simulink model "SVPWM_simscape"  (R2026a)
settings: Solver=ode23t  StartTime=1  StopTime=2  FixedStep=1e-7  RelTol=1e-5  AbsTol=1e-10
undefined symbols (not defined in the file): Down, PermanentMagnetSynchrono_class, Up
libraries: fl_lib x24, nesl_utility x20, ee_lib x8, eeTransforms x4, eePwmGenerator x3, simulink x3, elec_conv_HighZElecRef x2
(part 1 of 2)
settings Model: SimulationMode=accelerator  Creator=刘炳宏  LastModifiedBy=mushen
settings DebuggingCC: SaveWithParameterizedLinksMsg=none
settings SimscapeCC: SimscapeLogType=none  SimscapeLogDataHistory=5000.0

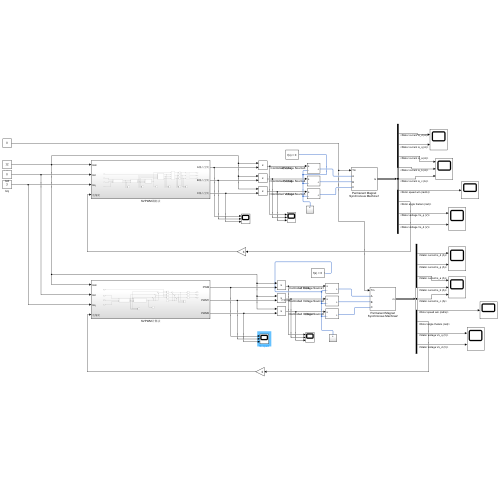
[thumbnail: Simulink's stored preview of the top-level diagram]
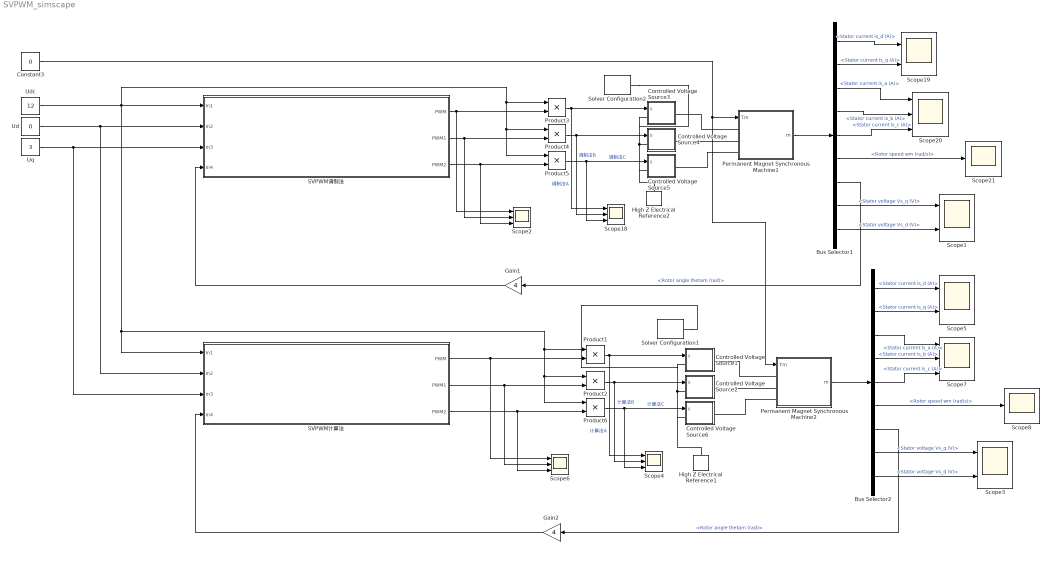
== system SVPWM_simscape ==
  Bus Selector1 : BusSelector  OutputSignals=Stator current is_d (A),Stator current is_q (A),Stator current is_a (A),Stator current is_b (A),Stator current is_c (A),Rotor speed wm (rad/s),Rotor angle thetam (rad),Stator voltage Vs_q (V),Stator voltage Vs_d (V)
  Bus Selector2 : BusSelector  OutputSignals=Stator current is_d (A),Stator current is_q (A),Stator current is_a (A),Stator current is_b (A),Stator current is_c (A),Rotor speed wm (rad/s),Rotor angle thetam (rad),Stator voltage Vs_q (V),Stator voltage Vs_d (V)
  Constant3 : Constant  Value=0
  Controlled Voltage Source1 : Subsystem
      settings: OpenFcn=elec.conv.unmask(gcb);
  Controlled Voltage Source2 : Subsystem
      settings: OpenFcn=elec.conv.unmask(gcb);
  Controlled Voltage Source3 : Subsystem
      settings: OpenFcn=elec.conv.unmask(gcb);
  Controlled Voltage Source4 : Subsystem
      settings: OpenFcn=elec.conv.unmask(gcb);
  Controlled Voltage Source5 : Subsystem
      settings: OpenFcn=elec.conv.unmask(gcb);
  Controlled Voltage Source6 : Subsystem
      settings: OpenFcn=elec.conv.unmask(gcb);
  Gain1 : Gain  Gain=4
  Gain2 : Gain  Gain=4
  High Z Electrical Reference1 : elec_conv_HighZElecRef/High Z Electrical Reference  SystemSampleTime=-1  VariantActivationTime=update diagram  EmptyChoice=off  PassThrough=off  PassThroughVariantControl=(default)  EmptyChoiceVariantControl=(default)  AllowFlexibleInterface=on  Latency=0  AutoFrameSizeCalculation=off
  High Z Electrical Reference2 : elec_conv_HighZElecRef/High Z Electrical Reference  SystemSampleTime=-1  VariantActivationTime=update diagram  EmptyChoice=off  PassThrough=off  PassThroughVariantControl=(default)  EmptyChoiceVariantControl=(default)  AllowFlexibleInterface=on  Latency=0  AutoFrameSizeCalculation=off
  Permanent Magnet Synchronous Machine1 : Subsystem
      settings: OpenFcn=elec.conv.unmask(gcb);
  Permanent Magnet Synchronous Machine2 : Subsystem
      settings: OpenFcn=elec.conv.unmask(gcb);
  Product{1..6} (6 alike) : Product
  SVPWM计算法 : Subsystem
  SVPWM调制法 : Subsystem
  Scope{1,3,5,19} (4 alike) : Scope  NumInputPorts=2
      Scope1 settings: ActiveDisplayYMinimum=-0.375  ActiveDisplayYMaximum=3.375
      Scope19 settings: ActiveDisplayYMinimum=-2.03311  ActiveDisplayYMaximum=2.45595  DataLoggingVariableName=ScopeData9
      Scope3 settings: ActiveDisplayYMinimum=-0.375  ActiveDisplayYMaximum=3.375  DataLoggingVariableName=ScopeData5
      Scope5 settings: ActiveDisplayYMinimum=-1.22545  ActiveDisplayYMaximum=3.73742  DataLoggingVariableName=ScopeData7
  Scope{2,4,6..7,18,20} (6 alike) : Scope  NumInputPorts=3
      Scope18 settings: ActiveDisplayYMinimum=2.7524  ActiveDisplayYMaximum=9.2476  DataLoggingVariableName=ScopeData8
      Scope2 settings: ActiveDisplayYMinimum=0.22937  ActiveDisplayYMaximum=0.77063
      Scope20 settings: ActiveDisplayYMinimum=-2.08518  ActiveDisplayYMaximum=2.2657  DataLoggingVariableName=ScopeData10
      Scope4 settings: ActiveDisplayYMinimum=-1.5  ActiveDisplayYMaximum=13.5  DataLoggingVariableName=ScopeData6
      Scope6 settings: ActiveDisplayYMinimum=0.22936706131906309  ActiveDisplayYMaximum=0.770632938680937  DataLoggingVariableName=ScopeData8
      Scope7 settings: ActiveDisplayYMinimum=-10.80387  ActiveDisplayYMaximum=10.80369  DataLoggingVariableName=ScopeData9
  Scope21 : Scope
      settings: ActiveDisplayYMinimum=-17.67923  ActiveDisplayYMaximum=27.92177  DataLoggingVariableName=ScopeData11
  Scope8 : Scope
      settings: ActiveDisplayYMinimum=-2.22769  ActiveDisplayYMaximum=20.0492  DataLoggingVariableName=ScopeData10
  Solver Configuration1 : nesl_utility/Solver Configuration  PhysicalDomain=network_engine_domain  SubClassName=solver  LeftPortType=input  RightPortType=generic  Tones=[]  Harmonics=[]  SimulateNoise=off  Profile=off  UseLocalSampling=off  EnableSwitchedLinearOptims=on  FrequencyDomain=off  UseCCode=off  RelTol=0.001  AbsTol=0.001  MinStep=1e-09  ToWorkspace=off  RevertToSquareIcSolve=off  NumHomotopyIterations=100  PhasorMode=off  PhasorModeNumHarmonics=1  ConsistencySolver=NEWTON_XTOL_AFTER_FTOL  CanonicalOrdering=CANONICAL  OptimizeIntermediates=OPTIMIZED  IndexReductionMethod=DerivativeReplacement  DoDC=off  ResidualTolerance=1e-09  ConsistencyTolSource=GLOBAL  ConsistencyAbsTol=0.001  ConsistencyRelTol=0.001  ConsistencyTolFactor=0.001  UseLocalSolver=off  LocalSolverChoice=NE_BACKWARD_EULER_ADVANCER  ResolveIndetEquations=on  FunctionEvalNumThread=1  LocalSolverSampleTime=0.001  DoFixedCost=off  MaxNonlinIter=3  MaxModeIter=2  ComputeImpulses=off  ImpulseIterations=2  LinearAlgebra=auto  LinearAlgebraNumThread=0  EquationFormulation=NE_TIME_EF  DelaysMemoryBudget=1024  AutomaticFiltering=on  FilteringTimeConstant=0.001  PartitionStorageMethod=AS_NEEDED  PartitionMemoryBudget=1024  PartitionMethod=ROBUST  MultibodyUseLocalSolver=off  MultibodyLocalSolverChoice=ODE1  MultibodyLocalSolverSampleTime=0.001
  Solver Configuration2 : nesl_utility/Solver Configuration  PhysicalDomain=network_engine_domain  SubClassName=solver  LeftPortType=input  RightPortType=generic  Tones=[]  Harmonics=[]  SimulateNoise=off  Profile=off  UseLocalSampling=off  EnableSwitchedLinearOptims=on  FrequencyDomain=off  UseCCode=off  RelTol=0.001  AbsTol=0.001  MinStep=1e-09  ToWorkspace=off  RevertToSquareIcSolve=off  NumHomotopyIterations=100  PhasorMode=off  PhasorModeNumHarmonics=1  ConsistencySolver=NEWTON_XTOL_AFTER_FTOL  CanonicalOrdering=CANONICAL  OptimizeIntermediates=OPTIMIZED  IndexReductionMethod=DerivativeReplacement  DoDC=off  ResidualTolerance=1e-09  ConsistencyTolSource=GLOBAL  ConsistencyAbsTol=0.001  ConsistencyRelTol=0.001  ConsistencyTolFactor=0.001  UseLocalSolver=off  LocalSolverChoice=NE_BACKWARD_EULER_ADVANCER  ResolveIndetEquations=on  FunctionEvalNumThread=1  LocalSolverSampleTime=0.001  DoFixedCost=off  MaxNonlinIter=3  MaxModeIter=2  ComputeImpulses=off  ImpulseIterations=2  LinearAlgebra=auto  LinearAlgebraNumThread=0  EquationFormulation=NE_TIME_EF  DelaysMemoryBudget=1024  AutomaticFiltering=on  FilteringTimeConstant=0.001  PartitionStorageMethod=AS_NEEDED  PartitionMemoryBudget=1024  PartitionMethod=ROBUST  MultibodyUseLocalSolver=off  MultibodyLocalSolverChoice=ODE1  MultibodyLocalSolverSampleTime=0.001
  Ud : Constant  Value=0
  Udc : Constant  Value=12
  Uq : Constant  Value=3
  wires:
  Product3/1 -> Controlled Voltage Source3/1(s), Scope18/1  "调制法A"
  Product4/1 -> Controlled Voltage Source4/1(s), Scope18/2  "调制法B"
  Product5/1 -> Controlled Voltage Source5/1(s), Scope18/3  "调制法C"
  Bus Selector1/7 -> Gain1/1  "<Rotor angle thetam (rad)>"
  Bus Selector1/5 -> Scope20/3  "<Stator current is_c (A)>"
  Bus Selector1/3 -> Scope20/1  "<Stator current is_a (A)>"
  Permanent Magnet Synchronous Machine1/1(m) -> Bus Selector1/1
  Bus Selector1/2 -> Scope19/2  "<Stator current is_q (A)>"
  Bus Selector1/6 -> Scope21/1  "<Rotor speed wm (rad/s)>"
  Bus Selector1/4 -> Scope20/2  "<Stator current is_b (A)>"
  Bus Selector1/1 -> Scope19/1  "<Stator current is_d (A)>"
  Bus Selector1/8 -> Scope1/1  "<Stator voltage Vs_q (V)>"
  Bus Selector1/9 -> Scope1/2  "<Stator voltage Vs_d (V)>"
  Constant3/1 -> Permanent Magnet Synchronous Machine1/1(Tm), Permanent Magnet Synchronous Machine2/1(Tm)
  Ud/1 -> SVPWM计算法/2(In2), SVPWM调制法/2(In2)
  Uq/1 -> SVPWM计算法/3(In3), SVPWM调制法/3(In3)
  SVPWM调制法/1(PWM) -> Scope2/1, Product3/2
  SVPWM调制法/2(PWM1) -> Scope2/2, Product4/2
  SVPWM调制法/3(PWM2) -> Scope2/3, Product5/2
  SVPWM计算法/1(PWM) -> Scope6/1, Product1/2
  SVPWM计算法/2(PWM1) -> Scope6/2, Product2/2
  Product6/1 -> Controlled Voltage Source6/1(s), Scope4/3  "计算法C"
  Product2/1 -> Controlled Voltage Source2/1(s), Scope4/2  "计算法B"
  Permanent Magnet Synchronous Machine2/1(m) -> Bus Selector2/1
  Bus Selector2/2 -> Scope5/2  "<Stator current is_q (A)>"
  Udc/1 -> Product2/1, Product6/1, Product1/1, SVPWM计算法/1(In1), Product4/1, Product5/1, Product3/1, SVPWM调制法/1(In1)
  Bus Selector2/4 -> Scope7/2  "<Stator current is_b (A)>"
  Bus Selector2/7 -> Gain2/1  "<Rotor angle thetam (rad)>"
  Bus Selector2/8 -> Scope3/1  "<Stator voltage Vs_q (V)>"
  Bus Selector2/9 -> Scope3/2  "<Stator voltage Vs_d (V)>"
  Bus Selector2/5 -> Scope7/3  "<Stator current is_c (A)>"
  SVPWM计算法/3(PWM2) -> Scope6/3, Product6/2
  Bus Selector2/1 -> Scope5/1  "<Stator current is_d (A)>"
  Bus Selector2/3 -> Scope7/1  "<Stator current is_a (A)>"
  Bus Selector2/6 -> Scope8/1  "<Rotor speed wm (rad/s)>"
  Product1/1 -> Controlled Voltage Source1/1(s), Scope4/1  "计算法A"
  Gain2/1 -> SVPWM计算法/4(In4)
  Gain1/1 -> SVPWM调制法/4(In4)
  connections:
  Controlled Voltage Source5/LConn1 -- High Z Electrical Reference2/LConn1 -- Solver Configuration2/RConn1 -- Controlled Voltage Source3/LConn1 -- Controlled Voltage Source4/LConn1
  Permanent Magnet Synchronous Machine1/LConn3 -- Controlled Voltage Source5/RConn1
  Permanent Magnet Synchronous Machine1/LConn1 -- Controlled Voltage Source3/RConn1
  Permanent Magnet Synchronous Machine1/LConn2 -- Controlled Voltage Source4/RConn1
  Controlled Voltage Source2/LConn1 -- Controlled Voltage Source1/LConn1 -- Solver Configuration1/RConn1 -- Controlled Voltage Source6/LConn1 -- High Z Electrical Reference1/LConn1
  Permanent Magnet Synchronous Machine2/LConn1 -- Controlled Voltage Source1/RConn1
  Permanent Magnet Synchronous Machine2/LConn3 -- Controlled Voltage Source6/RConn1
  Controlled Voltage Source2/RConn1 -- Permanent Magnet Synchronous Machine2/LConn2

== system SVPWM_simscape/Controlled Voltage Source1 ==
  s : Inport
  Controlled Voltage Source : fl_lib/Electrical/Electrical Sources/Controlled Voltage Source
  Simulink-PS Converter : nesl_utility/Simulink-PS Converter  PhysicalDomain=network_engine_domain  SubClassName=ps_input  LeftPortType=input  RightPortType=output  PseudoPeriodic=off  Frequencies=[]  NoiseDistribution=none  NoiseParameters=[]  Unit=1  AffineConversion=off  FilteringAndDerivatives=provide  SimscapeFilterOrder=1  InputFilterTimeConstant=0.001  UdotUserProvided=0
  - : PMIOPort  Side=Left
  + : PMIOPort  Port=2  Side=Right
  wires:
  s/1 -> Simulink-PS Converter/1
  connections:
  -/RConn1 -- Controlled Voltage Source/RConn2
  Simulink-PS Converter/RConn1 -- Controlled Voltage Source/RConn1
  Controlled Voltage Source/LConn1 -- +/RConn1

== system SVPWM_simscape/Controlled Voltage Source2 ==
  s : Inport
  Controlled Voltage Source : fl_lib/Electrical/Electrical Sources/Controlled Voltage Source
  Simulink-PS Converter : nesl_utility/Simulink-PS Converter  PhysicalDomain=network_engine_domain  SubClassName=ps_input  LeftPortType=input  RightPortType=output  PseudoPeriodic=off  Frequencies=[]  NoiseDistribution=none  NoiseParameters=[]  Unit=1  AffineConversion=off  FilteringAndDerivatives=provide  SimscapeFilterOrder=1  InputFilterTimeConstant=0.001  UdotUserProvided=0
  - : PMIOPort  Side=Left
  + : PMIOPort  Port=2  Side=Right
  wires:
  s/1 -> Simulink-PS Converter/1
  connections:
  -/RConn1 -- Controlled Voltage Source/RConn2
  Simulink-PS Converter/RConn1 -- Controlled Voltage Source/RConn1
  Controlled Voltage Source/LConn1 -- +/RConn1

== system SVPWM_simscape/Controlled Voltage Source3 ==
  s : Inport
  Controlled Voltage Source : fl_lib/Electrical/Electrical Sources/Controlled Voltage Source
  Simulink-PS Converter : nesl_utility/Simulink-PS Converter  PhysicalDomain=network_engine_domain  SubClassName=ps_input  LeftPortType=input  RightPortType=output  PseudoPeriodic=off  Frequencies=[]  NoiseDistribution=none  NoiseParameters=[]  Unit=1  AffineConversion=off  FilteringAndDerivatives=provide  SimscapeFilterOrder=1  InputFilterTimeConstant=0.001  UdotUserProvided=0
  - : PMIOPort  Side=Left
  + : PMIOPort  Port=2  Side=Right
  wires:
  s/1 -> Simulink-PS Converter/1
  connections:
  -/RConn1 -- Controlled Voltage Source/RConn2
  Simulink-PS Converter/RConn1 -- Controlled Voltage Source/RConn1
  Controlled Voltage Source/LConn1 -- +/RConn1

== system SVPWM_simscape/Controlled Voltage Source4 ==
  s : Inport
  Controlled Voltage Source : fl_lib/Electrical/Electrical Sources/Controlled Voltage Source
  Simulink-PS Converter : nesl_utility/Simulink-PS Converter  PhysicalDomain=network_engine_domain  SubClassName=ps_input  LeftPortType=input  RightPortType=output  PseudoPeriodic=off  Frequencies=[]  NoiseDistribution=none  NoiseParameters=[]  Unit=1  AffineConversion=off  FilteringAndDerivatives=provide  SimscapeFilterOrder=1  InputFilterTimeConstant=0.001  UdotUserProvided=0
  - : PMIOPort  Side=Left
  + : PMIOPort  Port=2  Side=Right
  wires:
  s/1 -> Simulink-PS Converter/1
  connections:
  -/RConn1 -- Controlled Voltage Source/RConn2
  Simulink-PS Converter/RConn1 -- Controlled Voltage Source/RConn1
  Controlled Voltage Source/LConn1 -- +/RConn1

== system SVPWM_simscape/Controlled Voltage Source5 ==
  s : Inport
  Controlled Voltage Source : fl_lib/Electrical/Electrical Sources/Controlled Voltage Source
  Simulink-PS Converter : nesl_utility/Simulink-PS Converter  PhysicalDomain=network_engine_domain  SubClassName=ps_input  LeftPortType=input  RightPortType=output  PseudoPeriodic=off  Frequencies=[]  NoiseDistribution=none  NoiseParameters=[]  Unit=1  AffineConversion=off  FilteringAndDerivatives=provide  SimscapeFilterOrder=1  InputFilterTimeConstant=0.001  UdotUserProvided=0
  - : PMIOPort  Side=Left
  + : PMIOPort  Port=2  Side=Right
  wires:
  s/1 -> Simulink-PS Converter/1
  connections:
  -/RConn1 -- Controlled Voltage Source/RConn2
  Simulink-PS Converter/RConn1 -- Controlled Voltage Source/RConn1
  Controlled Voltage Source/LConn1 -- +/RConn1

== system SVPWM_simscape/Controlled Voltage Source6 ==
  s : Inport
  Controlled Voltage Source : fl_lib/Electrical/Electrical Sources/Controlled Voltage Source
  Simulink-PS Converter : nesl_utility/Simulink-PS Converter  PhysicalDomain=network_engine_domain  SubClassName=ps_input  LeftPortType=input  RightPortType=output  PseudoPeriodic=off  Frequencies=[]  NoiseDistribution=none  NoiseParameters=[]  Unit=1  AffineConversion=off  FilteringAndDerivatives=provide  SimscapeFilterOrder=1  InputFilterTimeConstant=0.001  UdotUserProvided=0
  - : PMIOPort  Side=Left
  + : PMIOPort  Port=2  Side=Right
  wires:
  s/1 -> Simulink-PS Converter/1
  connections:
  -/RConn1 -- Controlled Voltage Source/RConn2
  Simulink-PS Converter/RConn1 -- Controlled Voltage Source/RConn1
  Controlled Voltage Source/LConn1 -- +/RConn1

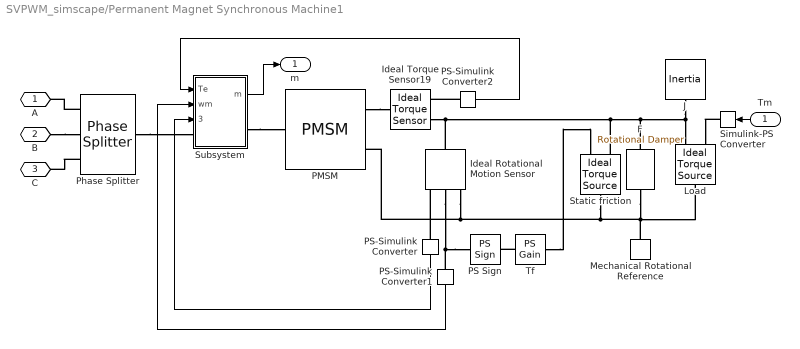
== system SVPWM_simscape/Permanent Magnet Synchronous Machine1 ==
  Tm : Inport
  F : fl_lib/Mechanical/Rotational Elements/Rotational Damper  D=0.0003505 N*m/(rad/s)  w_specify=on  w_priority=High  w=0 rad/s  w_nominal_specify=off  w_nominal_value=1  w_nominal_unit=rad/s  t_specify=off  t_priority=None  t=0 N*m  t_nominal_specify=off  t_nominal_value=1  t_nominal_unit=N*m
  Ideal Rotational Motion Sensor : fl_lib/Mechanical/Mechanical Sensors/Ideal Rotational Motion Sensor  reference=foundation.enum.MeasurementReference.difference  acceleration_port=false  velocity_port=true  position_port=true  wrap_angle=simscape.enum.onoff.off  offset=1 deg
  Ideal Torque Sensor19 : fl_lib/Mechanical/Mechanical Sensors/Ideal Torque Sensor
  J : fl_lib/Mechanical/Rotational Elements/Inertia  inertia=0.00062 kg*m^2  num_ports=foundation.enum.numPorts2.one  w_specify=on  w_priority=High  w=0 rad/s  w_nominal_specify=off  w_nominal_value=1  w_nominal_unit=rad/s  t_specify=off  t_priority=None  t=0 N*m  t_nominal_specify=off  t_nominal_value=1  t_nominal_unit=N*m
  Load : fl_lib/Mechanical/Mechanical Sources/Ideal Torque Source
  Mechanical Rotational Reference : fl_lib/Mechanical/Rotational Elements/Mechanical Rotational Reference
  PMSM : ee_lib/Electromechanical/Permanent Magnet/PMSM  port_option=ee.enum.threePhasePort.composite  winding_type=ee.enum.statorconnection.wye  machine_param=ee.enum.pmsm.parameterization.constant  nPolePairs=4  pmflux_param=1  pm_flux_linkage=PermanentMagnetSynchrono_class('Torque Tm',[0.00062 0.0003505 4 0],4,'Flux linkage established by magnets (V.s)',0.074147,53.7951,0.44488,'Aligned with phase A axis (original Park)',[0 1 0 0],'Sinusoidal',120,'3',[0 0 0 0 0 0]).objParamMappingDerived.NewDerivedParam.pm_flux_linkage Wb  torque_constant=0.18 N*m/A  back_emf_constant=0.18 V/(rad/s)  stator_param=1  Ld=0.0085 H  Lq=0.0085 H  idVec=[-200, 0, 200] A  iqVec=[-200, 0, 200] A  LdMatrix=0.0002 * ones(3, 3) H  LqMatrix=0.0002 * ones(3, 3) H  PmMatrix=0.1 * ones(3, 3) Wb  ktMatrix=0.18 * ones(3, 3) N*m/A  keMatrix=0.18 * ones(3, 3) V/(rad/s)  L0=1e-09 H  Ls=0.0002 H  Lm=-0.00002 H  Ms=0.00002 H  Rs=0.18 Ohm  zero_sequence=0  axes_param=2  loss_param=ee.enum.ironloss.none  losses_oc=[0, 0, 0] W  losses_sc=[0, 0, 0] W  f_losses=60 Hz  Isc_losses=95 A  J=0 kg*m^2  lam=0 N*m/(rad/s)  i_d_specify=on  i_d_priority=High  i_d=PermanentMagnetSynchrono_class('Torque Tm',[0.00062 0.0003505 4 0],4,'Flux linkage established by magnets (V.s)',0.074147,53.7951,0.44488,'Aligned with phase A axis (original Park)',[0 1 0 0],'Sinusoidal',120,'3',[0 0 0 0 0 0]).objParamMappingDerived.NewDerivedParam.i_d A  i_d_nominal_specify=off  i_d_nominal_value=1  i_d_nominal_unit=A  i_q_specify=on  i_q_priority=High  i_q=PermanentMagnetSynchrono_class('Torque Tm',[0.00062 0.0003505 4 0],4,'Flux linkage established by magnets (V.s)',0.074147,53.7951,0.44488,'Aligned with phase A axis (original Park)',[0 1 0 0],'Sinusoidal',120,'3',[0 0 0 0 0 0]).objParamMappingDerived.NewDerivedParam.i_q A  i_q_nominal_specify=off  i_q_nominal_value=1  i_q_nominal_unit=A  torque_specify=off  torque_priority=None  torque=0 N*m  torque_nominal_specify=off  torque_nominal_value=1  torque_nominal_unit=N*m  angular_velocity_specify=on  angular_velocity_priority=High  angular_velocity=0 rad/s  angular_velocity_nominal_specify=off  angular_velocity_nominal_value=1  angular_velocity_nominal_unit=rpm  angular_position_specify=on  angular_position_priority=High  angular_position=1 deg  angular_position_nominal_specify=off  angular_position_nominal_value=1  angular_position_nominal_unit=deg  alpha=3.93e-3 1/K  alpha_flux=-0.001 1/K  Tmeas=298.15 K  stator_thermal_mass=100 J/K  rotor_thermal_mass=200 J/K  Rm_percent_rotor=90  Rd_percent_rotor=30  temperatureA_specify=off  temperatureA_priority=High  temperatureA=25 degC  temperatureA_nominal_specify=off  temperatureA_nominal_value=1  temperatureA_nominal_unit=degC  temperatureB_specify=off  temperatureB_priority=High  temperatureB=25 degC  temperatureB_nominal_specify=off  temperatureB_nominal_value=1  temperatureB_nominal_unit=degC  temperatureC_specify=off  temperatureC_priority=High  temperatureC=25 degC  temperatureC_nominal_specify=off  temperatureC_nominal_value=1  temperatureC_nominal_unit=degC  temperatureR_specify=off  temperatureR_priority=High  temperatureR=25 degC  temperatureR_nominal_specify=off  temperatureR_nominal_value=1  temperatureR_nominal_unit=degC
  PS Sign : fl_lib/Physical Signals/Nonlinear Operators/PS Sign
  PS-Simulink Converter : nesl_utility/PS-Simulink Converter  PhysicalDomain=network_engine_domain  SubClassName=ps_output  LeftPortType=input  RightPortType=output  PseudoPeriodic=off  Frequencies=[]  VectorFormat=1-D array  Unit=1  AffineConversion=off
  PS-Simulink Converter1 : nesl_utility/PS-Simulink Converter  PhysicalDomain=network_engine_domain  SubClassName=ps_output  LeftPortType=input  RightPortType=output  PseudoPeriodic=off  Frequencies=[]  VectorFormat=1-D array  Unit=1  AffineConversion=off
  PS-Simulink Converter2 : nesl_utility/PS-Simulink Converter  PhysicalDomain=network_engine_domain  SubClassName=ps_output  LeftPortType=input  RightPortType=output  PseudoPeriodic=off  Frequencies=[]  VectorFormat=1-D array  Unit=1  AffineConversion=off
  Phase Splitter : ee_lib/Connectors & References/Phase Splitter
  Simulink-PS Converter : nesl_utility/Simulink-PS Converter  PhysicalDomain=network_engine_domain  SubClassName=ps_input  LeftPortType=input  RightPortType=output  PseudoPeriodic=off  Frequencies=[]  NoiseDistribution=none  NoiseParameters=[]  Unit=1  AffineConversion=off  FilteringAndDerivatives=provide  SimscapeFilterOrder=1  InputFilterTimeConstant=0.001  UdotUserProvided=0
  Static friction : fl_lib/Mechanical/Mechanical Sources/Ideal Torque Source
  Subsystem : Subsystem
  Tf : fl_lib/Physical Signals/Functions/PS Gain  gain=PermanentMagnetSynchrono_class('Torque Tm',[0.00062 0.0003505 4 0],4,'Flux linkage established by magnets (V.s)',0.074147,53.7951,0.44488,'Aligned with phase A axis (original Park)',[0 1 0 0],'Sinusoidal',120,'3',[0 0 0 0 0 0]).objParamMappingDerived.NewDerivedParam.Tf
  A : PMIOPort  Side=Left
  B : PMIOPort  Port=2  Side=Left
  C : PMIOPort  Port=3  Side=Left
  m : Outport  VectorParamsAs1DForOutWhenUnconnected=off
  wires:
  PS-Simulink Converter1/1 -> Subsystem/2(wm)
  PS-Simulink Converter/1 -> Subsystem/3(thetam)
  PS-Simulink Converter2/1 -> Subsystem/1(Te)
  Subsystem/1(m) -> m/1
  Tm/1 -> Simulink-PS Converter/1
  connections:
  PS-Simulink Converter2/LConn1 -- Ideal Torque Sensor19/RConn2
  Phase Splitter/LConn1 -- Subsystem/LConn1
  Subsystem/RConn1 -- PMSM/LConn1
  PS-Simulink Converter/LConn1 -- Ideal Rotational Motion Sensor/RConn3
  Tf/RConn1 -- Static friction/RConn1
  PS Sign/LConn1 -- PS-Simulink Converter1/LConn1 -- Ideal Rotational Motion Sensor/RConn2
  Tf/LConn1 -- PS Sign/RConn1
  PMSM/RConn1 -- Ideal Torque Sensor19/LConn1
  Ideal Torque Sensor19/RConn1 -- Static friction/RConn2 -- F/LConn1 -- Load/RConn2 -- J/LConn1 -- Ideal Rotational Motion Sensor/LConn1
  Phase Splitter/RConn3 -- C/RConn1
  Phase Splitter/RConn1 -- A/RConn1
  B/RConn1 -- Phase Splitter/RConn2
  Simulink-PS Converter/RConn1 -- Load/RConn1
  Load/LConn1 -- F/RConn1 -- Static friction/LConn1 -- PMSM/RConn2 -- Ideal Rotational Motion Sensor/RConn1 -- Mechanical Rotational Reference/LConn1

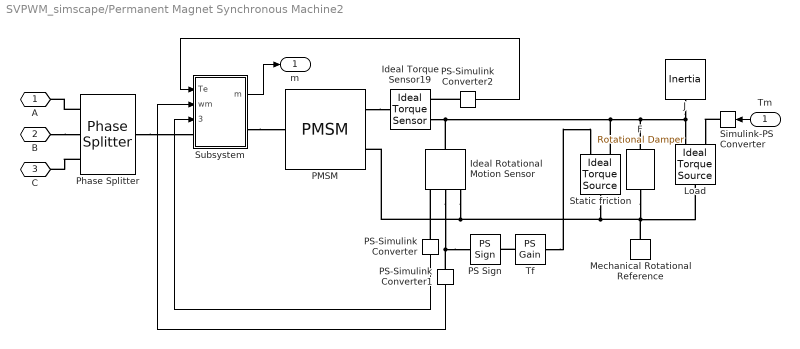
== system SVPWM_simscape/Permanent Magnet Synchronous Machine2 ==
  Tm : Inport
  F : fl_lib/Mechanical/Rotational Elements/Rotational Damper  D=0.0003505 N*m/(rad/s)  w_specify=on  w_priority=High  w=0 rad/s  w_nominal_specify=off  w_nominal_value=1  w_nominal_unit=rad/s  t_specify=off  t_priority=None  t=0 N*m  t_nominal_specify=off  t_nominal_value=1  t_nominal_unit=N*m
  Ideal Rotational Motion Sensor : fl_lib/Mechanical/Mechanical Sensors/Ideal Rotational Motion Sensor  reference=foundation.enum.MeasurementReference.difference  acceleration_port=false  velocity_port=true  position_port=true  wrap_angle=simscape.enum.onoff.off  offset=1 deg
  Ideal Torque Sensor19 : fl_lib/Mechanical/Mechanical Sensors/Ideal Torque Sensor
  J : fl_lib/Mechanical/Rotational Elements/Inertia  inertia=0.00062 kg*m^2  num_ports=foundation.enum.numPorts2.one  w_specify=on  w_priority=High  w=0 rad/s  w_nominal_specify=off  w_nominal_value=1  w_nominal_unit=rad/s  t_specify=off  t_priority=None  t=0 N*m  t_nominal_specify=off  t_nominal_value=1  t_nominal_unit=N*m
  Load : fl_lib/Mechanical/Mechanical Sources/Ideal Torque Source
  Mechanical Rotational Reference : fl_lib/Mechanical/Rotational Elements/Mechanical Rotational Reference
  PMSM : ee_lib/Electromechanical/Permanent Magnet/PMSM  port_option=ee.enum.threePhasePort.composite  winding_type=ee.enum.statorconnection.wye  machine_param=ee.enum.pmsm.parameterization.constant  nPolePairs=4  pmflux_param=1  pm_flux_linkage=PermanentMagnetSynchrono_class('Torque Tm',[0.00062 0.0003505 4 0],4,'Flux linkage established by magnets (V.s)',0.074147,53.7951,0.44488,'Aligned with phase A axis (original Park)',[0 1 0 0],'Sinusoidal',120,'3',[0 0 0 0 0 0]).objParamMappingDerived.NewDerivedParam.pm_flux_linkage Wb  torque_constant=0.18 N*m/A  back_emf_constant=0.18 V/(rad/s)  stator_param=1  Ld=0.0085 H  Lq=0.0085 H  idVec=[-200, 0, 200] A  iqVec=[-200, 0, 200] A  LdMatrix=0.0002 * ones(3, 3) H  LqMatrix=0.0002 * ones(3, 3) H  PmMatrix=0.1 * ones(3, 3) Wb  ktMatrix=0.18 * ones(3, 3) N*m/A  keMatrix=0.18 * ones(3, 3) V/(rad/s)  L0=1e-09 H  Ls=0.0002 H  Lm=-0.00002 H  Ms=0.00002 H  Rs=0.18 Ohm  zero_sequence=0  axes_param=2  loss_param=ee.enum.ironloss.none  losses_oc=[0, 0, 0] W  losses_sc=[0, 0, 0] W  f_losses=60 Hz  Isc_losses=95 A  J=0 kg*m^2  lam=0 N*m/(rad/s)  i_d_specify=on  i_d_priority=High  i_d=PermanentMagnetSynchrono_class('Torque Tm',[0.00062 0.0003505 4 0],4,'Flux linkage established by magnets (V.s)',0.074147,53.7951,0.44488,'Aligned with phase A axis (original Park)',[0 1 0 0],'Sinusoidal',120,'3',[0 0 0 0 0 0]).objParamMappingDerived.NewDerivedParam.i_d A  i_d_nominal_specify=off  i_d_nominal_value=1  i_d_nominal_unit=A  i_q_specify=on  i_q_priority=High  i_q=PermanentMagnetSynchrono_class('Torque Tm',[0.00062 0.0003505 4 0],4,'Flux linkage established by magnets (V.s)',0.074147,53.7951,0.44488,'Aligned with phase A axis (original Park)',[0 1 0 0],'Sinusoidal',120,'3',[0 0 0 0 0 0]).objParamMappingDerived.NewDerivedParam.i_q A  i_q_nominal_specify=off  i_q_nominal_value=1  i_q_nominal_unit=A  torque_specify=off  torque_priority=None  torque=0 N*m  torque_nominal_specify=off  torque_nominal_value=1  torque_nominal_unit=N*m  angular_velocity_specify=on  angular_velocity_priority=High  angular_velocity=0 rad/s  angular_velocity_nominal_specify=off  angular_velocity_nominal_value=1  angular_velocity_nominal_unit=rpm  angular_position_specify=on  angular_position_priority=High  angular_position=1 deg  angular_position_nominal_specify=off  angular_position_nominal_value=1  angular_position_nominal_unit=deg  alpha=3.93e-3 1/K  alpha_flux=-0.001 1/K  Tmeas=298.15 K  stator_thermal_mass=100 J/K  rotor_thermal_mass=200 J/K  Rm_percent_rotor=90  Rd_percent_rotor=30  temperatureA_specify=off  temperatureA_priority=High  temperatureA=25 degC  temperatureA_nominal_specify=off  temperatureA_nominal_value=1  temperatureA_nominal_unit=degC  temperatureB_specify=off  temperatureB_priority=High  temperatureB=25 degC  temperatureB_nominal_specify=off  temperatureB_nominal_value=1  temperatureB_nominal_unit=degC  temperatureC_specify=off  temperatureC_priority=High  temperatureC=25 degC  temperatureC_nominal_specify=off  temperatureC_nominal_value=1  temperatureC_nominal_unit=degC  temperatureR_specify=off  temperatureR_priority=High  temperatureR=25 degC  temperatureR_nominal_specify=off  temperatureR_nominal_value=1  temperatureR_nominal_unit=degC
  PS Sign : fl_lib/Physical Signals/Nonlinear Operators/PS Sign
  PS-Simulink Converter : nesl_utility/PS-Simulink Converter  PhysicalDomain=network_engine_domain  SubClassName=ps_output  LeftPortType=input  RightPortType=output  PseudoPeriodic=off  Frequencies=[]  VectorFormat=1-D array  Unit=1  AffineConversion=off
  PS-Simulink Converter1 : nesl_utility/PS-Simulink Converter  PhysicalDomain=network_engine_domain  SubClassName=ps_output  LeftPortType=input  RightPortType=output  PseudoPeriodic=off  Frequencies=[]  VectorFormat=1-D array  Unit=1  AffineConversion=off
  PS-Simulink Converter2 : nesl_utility/PS-Simulink Converter  PhysicalDomain=network_engine_domain  SubClassName=ps_output  LeftPortType=input  RightPortType=output  PseudoPeriodic=off  Frequencies=[]  VectorFormat=1-D array  Unit=1  AffineConversion=off
  Phase Splitter : ee_lib/Connectors & References/Phase Splitter
  Simulink-PS Converter : nesl_utility/Simulink-PS Converter  PhysicalDomain=network_engine_domain  SubClassName=ps_input  LeftPortType=input  RightPortType=output  PseudoPeriodic=off  Frequencies=[]  NoiseDistribution=none  NoiseParameters=[]  Unit=1  AffineConversion=off  FilteringAndDerivatives=provide  SimscapeFilterOrder=1  InputFilterTimeConstant=0.001  UdotUserProvided=0
  Static friction : fl_lib/Mechanical/Mechanical Sources/Ideal Torque Source
  Subsystem : Subsystem
  Tf : fl_lib/Physical Signals/Functions/PS Gain  gain=PermanentMagnetSynchrono_class('Torque Tm',[0.00062 0.0003505 4 0],4,'Flux linkage established by magnets (V.s)',0.074147,53.7951,0.44488,'Aligned with phase A axis (original Park)',[0 1 0 0],'Sinusoidal',120,'3',[0 0 0 0 0 0]).objParamMappingDerived.NewDerivedParam.Tf
  A : PMIOPort  Side=Left
  B : PMIOPort  Port=2  Side=Left
  C : PMIOPort  Port=3  Side=Left
  m : Outport  VectorParamsAs1DForOutWhenUnconnected=off
  wires:
  PS-Simulink Converter1/1 -> Subsystem/2(wm)
  PS-Simulink Converter/1 -> Subsystem/3(thetam)
  PS-Simulink Converter2/1 -> Subsystem/1(Te)
  Subsystem/1(m) -> m/1
  Tm/1 -> Simulink-PS Converter/1
  connections:
  PS-Simulink Converter2/LConn1 -- Ideal Torque Sensor19/RConn2
  Phase Splitter/LConn1 -- Subsystem/LConn1
  Subsystem/RConn1 -- PMSM/LConn1
  PS-Simulink Converter/LConn1 -- Ideal Rotational Motion Sensor/RConn3
  Tf/RConn1 -- Static friction/RConn1
  PS Sign/LConn1 -- PS-Simulink Converter1/LConn1 -- Ideal Rotational Motion Sensor/RConn2
  Tf/LConn1 -- PS Sign/RConn1
  PMSM/RConn1 -- Ideal Torque Sensor19/LConn1
  Ideal Torque Sensor19/RConn1 -- Static friction/RConn2 -- F/LConn1 -- Load/RConn2 -- J/LConn1 -- Ideal Rotational Motion Sensor/LConn1
  Phase Splitter/RConn3 -- C/RConn1
  Phase Splitter/RConn1 -- A/RConn1
  B/RConn1 -- Phase Splitter/RConn2
  Simulink-PS Converter/RConn1 -- Load/RConn1
  Load/LConn1 -- F/RConn1 -- Static friction/LConn1 -- PMSM/RConn2 -- Ideal Rotational Motion Sensor/RConn1 -- Mechanical Rotational Reference/LConn1

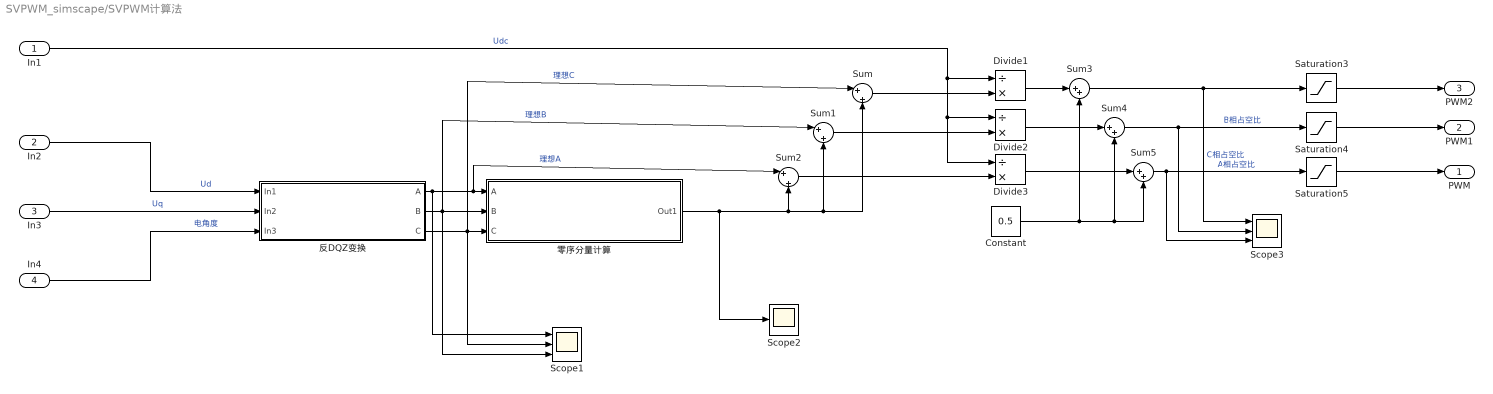
== system SVPWM_simscape/SVPWM计算法 ==
  In1 : Inport
  In2 : Inport  Port=2
  In3 : Inport  Port=3
  In4 : Inport  Port=4
  Constant : Constant  Value=0.5
  Divide1 : Product  Inputs=/*
  Divide2 : Product  Inputs=/*
  Divide3 : Product  Inputs=/*
  Saturation3 : Saturate  UpperLimit=1  LowerLimit=0
  Saturation4 : Saturate  UpperLimit=1  LowerLimit=0
  Saturation5 : Saturate  UpperLimit=1  LowerLimit=0
  Scope1 : Scope  NumInputPorts=3
      settings: ActiveDisplayYMinimum=-3.13505  ActiveDisplayYMaximum=3.34432  DataLoggingVariableName=ScopeData2
  Scope2 : Scope
      settings: ActiveDisplayYMinimum=-0.20463  ActiveDisplayYMaximum=-0.00463  DataLoggingVariableName=ScopeData4
  Scope3 : Scope  NumInputPorts=3
      settings: ActiveDisplayYMinimum=0.23003  ActiveDisplayYMaximum=0.76997  DataLoggingVariableName=ScopeData3
  Sum : Sum  Inputs=|+|+
  Sum1 : Sum  Inputs=|+|+
  Sum2 : Sum  Inputs=|+|+
  Sum3 : Sum  Inputs=|++
  Sum4 : Sum  Inputs=|++
  Sum5 : Sum  Inputs=|++
  反DQZ变换 : Subsystem
  零序分量计算 : Subsystem
  PWM : Outport
  PWM1 : Outport  Port=2
  PWM2 : Outport  Port=3
  wires:
  Sum5/1 -> Scope3/3, Saturation5/1  "A相占空比"
  Sum4/1 -> Saturation4/1, Scope3/2  "B相占空比"
  In3/1 -> 反DQZ变换/2(In2)  "Uq"
  In4/1 -> 反DQZ变换/3(In3)  "电角度"
  Sum3/1 -> Scope3/1, Saturation3/1  "C相占空比"
  In2/1 -> 反DQZ变换/1(In1)  "Ud"
  反DQZ变换/1(A) -> Sum2/1, 零序分量计算/1(A), Scope1/1  "理想A"
  反DQZ变换/2(B) -> Sum1/1, Scope1/3, 零序分量计算/2(B)  "理想B"
  反DQZ变换/3(C) -> Sum/1, Scope1/2, 零序分量计算/3(C)  "理想C"
  零序分量计算/1(Out1) -> Sum2/2, Sum/2, Sum1/2, Scope2/1
  Sum2/1 -> Divide3/2
  Sum1/1 -> Divide2/2
  Sum/1 -> Divide1/2
  In1/1 -> Divide3/1, Divide2/1, Divide1/1  "Udc"
  Divide1/1 -> Sum3/1
  Divide3/1 -> Sum5/1
  Divide2/1 -> Sum4/1
  Constant/1 -> Sum3/2, Sum4/2, Sum5/2
  Saturation4/1 -> PWM1/1
  Saturation3/1 -> PWM2/1
  Saturation5/1 -> PWM/1

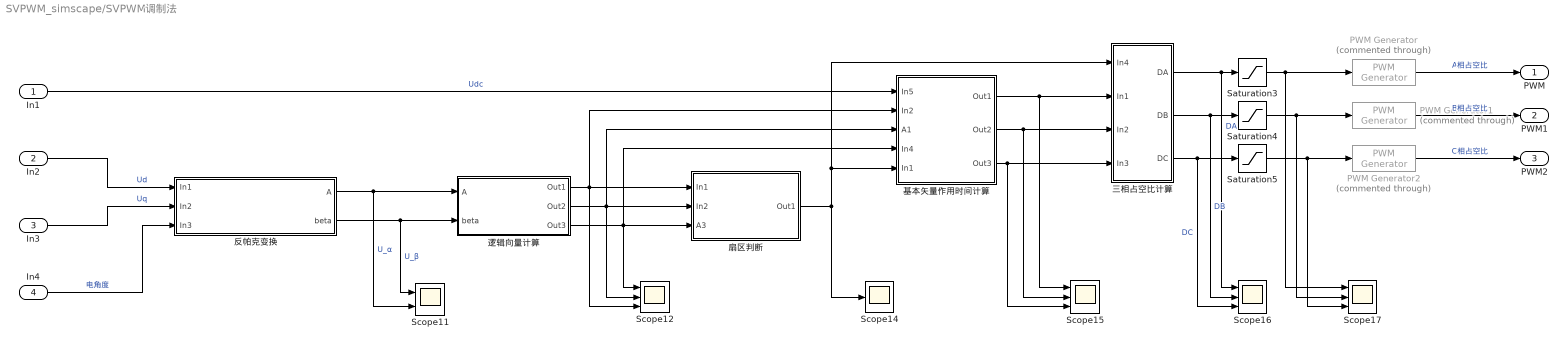
== system SVPWM_simscape/SVPWM调制法 ==
  In1 : Inport
  In2 : Inport  Port=2
  In3 : Inport  Port=3
  In4 : Inport  Port=4
  PWM Generator : eePwmGenerator/PWM Generator  Commented=through  CarrCount=Up-Down  Tper=1/16000  Tdelay=0  Ts=5e-6
  PWM Generator1 : eePwmGenerator/PWM Generator  Commented=through  CarrCount=Up-Down  Tper=1/16000  Tdelay=0  Ts=5e-6
  PWM Generator2 : eePwmGenerator/PWM Generator  Commented=through  CarrCount=Up-Down  Tper=1/16000  Tdelay=0  Ts=5e-6
  Saturation3 : Saturate  UpperLimit=1  LowerLimit=0
  Saturation4 : Saturate  UpperLimit=1  LowerLimit=0
  Saturation5 : Saturate  UpperLimit=1  LowerLimit=0
  Scope11 : Scope  NumInputPorts=2
      settings: SampleTime=0.00001  ActiveDisplayYMinimum=-1.82854  ActiveDisplayYMaximum=10.17881
  Scope{12,15..17} (4 alike) : Scope  NumInputPorts=3
      Scope12 settings: ActiveDisplayYMinimum=-6.25  ActiveDisplayYMaximum=6.25  DataLoggingVariableName=ScopeData2
      Scope15 settings: ActiveDisplayYMinimum=-0.09375  ActiveDisplayYMaximum=0.84375  DataLoggingVariableName=ScopeData5
      Scope16 settings: ActiveDisplayYMinimum=0.22937  ActiveDisplayYMaximum=0.77063  DataLoggingVariableName=ScopeData6
      Scope17 settings: ActiveDisplayYMinimum=0.43459  ActiveDisplayYMaximum=1.06282  DataLoggingVariableName=ScopeData7
  Scope14 : Scope
      settings: ActiveDisplayYMinimum=0.375  ActiveDisplayYMaximum=6.625  DataLoggingVariableName=ScopeData4
  三相占空比计算 : Subsystem
  反帕克变换 : Subsystem
  基本矢量作用时间计算 : Subsystem
  扇区判断 : Subsystem
  逻辑向量计算 : Subsystem
  PWM : Outport
  PWM1 : Outport  Port=2
  PWM2 : Outport  Port=3
  wires:
  Saturation4/1 -> PWM Generator1/1, Scope17/2
  逻辑向量计算/2(Out2) -> 基本矢量作用时间计算/3(A1), Scope12/2, 扇区判断/2(In2)
  三相占空比计算/3(DC) -> Scope16/3, Saturation5/1  "DC"
  PWM Generator/1 -> PWM/1  "A相占空比"
  基本矢量作用时间计算/1(Out1) -> 三相占空比计算/2(In1), Scope15/1
  反帕克变换/1(A) -> Scope11/2, 逻辑向量计算/1(A)  "U_α"
  基本矢量作用时间计算/3(Out3) -> 三相占空比计算/4(In3), Scope15/3
  基本矢量作用时间计算/2(Out2) -> 三相占空比计算/3(In2), Scope15/2
  Saturation3/1 -> Scope17/1, PWM Generator/1
  扇区判断/1(Out1) -> Scope14/1, 三相占空比计算/1(In4), 基本矢量作用时间计算/5(In1)
  三相占空比计算/2(DB) -> Scope16/2, Saturation4/1  "DB"
  PWM Generator1/1 -> PWM1/1  "B相占空比"
  反帕克变换/2(beta) -> Scope11/1, 逻辑向量计算/2(beta)  "U_β"
  三相占空比计算/1(DA) -> Scope16/1, Saturation3/1  "DA"
  Saturation5/1 -> PWM Generator2/1, Scope17/3
  逻辑向量计算/1(Out1) -> 扇区判断/1(In1), 基本矢量作用时间计算/2(In2), Scope12/3
  逻辑向量计算/3(Out3) -> 基本矢量作用时间计算/4(In4), Scope12/1, 扇区判断/3(A3)
  In3/1 -> 反帕克变换/2(In2)  "Uq"
  In4/1 -> 反帕克变换/3(In3)  "电角度"
  PWM Generator2/1 -> PWM2/1  "C相占空比"
  In1/1 -> 基本矢量作用时间计算/1(In5)  "Udc"
  In2/1 -> 反帕克变换/1(In1)  "Ud"

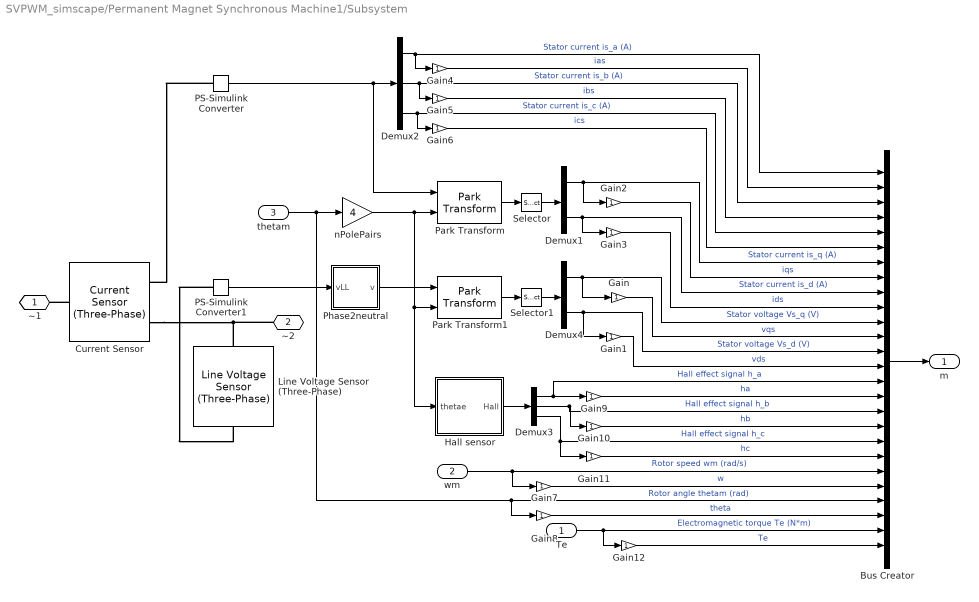
== system SVPWM_simscape/Permanent Magnet Synchronous Machine1/Subsystem ==
  Te : Inport
  wm : Inport  Port=2
  thetam : Inport  Port=3
  Bus Creator : BusCreator  Inputs=26
  Current Sensor : ee_lib/Sensors & Transducers/Current Sensor (Three-Phase)  port_option=ee.enum.threePhasePort.composite
  Demux1 : Demux  Outputs=2
  Demux2 : Demux  Outputs=3
  Demux3 : Demux  Outputs=3
  Demux4 : Demux  Outputs=2
  Gain{,1..12} (13 alike) : Gain
  Hall sensor : Subsystem
  Line Voltage Sensor (Three-Phase) : ee_lib/Sensors & Transducers/Line Voltage Sensor (Three-Phase)  port_option=ee.enum.threePhasePort.composite
  PS-Simulink Converter : nesl_utility/PS-Simulink Converter  PhysicalDomain=network_engine_domain  SubClassName=ps_output  LeftPortType=input  RightPortType=output  PseudoPeriodic=off  Frequencies=[]  VectorFormat=1-D array  Unit=1  AffineConversion=off
  PS-Simulink Converter1 : nesl_utility/PS-Simulink Converter  PhysicalDomain=network_engine_domain  SubClassName=ps_output  LeftPortType=input  RightPortType=output  PseudoPeriodic=off  Frequencies=[]  VectorFormat=1-D array  Unit=1  AffineConversion=off
  Park Transform : eeTransforms/Park Transform  AxisAlignment=D-axis  PowerInvariant=off
  Park Transform1 : eeTransforms/Park Transform  AxisAlignment=D-axis  PowerInvariant=off
  Phase2neutral : Subsystem
  Selector : Selector  InputPortWidth=3  IndexOptions=Index vector (dialog)  Indices=[2 1]  OutputSizes=1
  Selector1 : Selector  InputPortWidth=3  IndexOptions=Index vector (dialog)  Indices=[2 1]  OutputSizes=1
  nPolePairs : Gain  Gain=4
  ~1 : PMIOPort  Side=Left
  ~2 : PMIOPort  Port=2  Side=Right
  m : Outport  VectorParamsAs1DForOutWhenUnconnected=off
  wires:
  Phase2neutral/1(v) -> Park Transform1/1
  Gain8/1 -> Bus Creator/24  "theta"
  Gain7/1 -> Bus Creator/22  "w"
  Selector1/1 -> Demux4/1
  Selector/1 -> Demux1/1
  Gain11/1 -> Bus Creator/20  "hc"
  Gain10/1 -> Bus Creator/18  "hb"
  Gain9/1 -> Bus Creator/16  "ha"
  Gain1/1 -> Bus Creator/14  "vds"
  Gain/1 -> Bus Creator/12  "vqs"
  Gain3/1 -> Bus Creator/10  "ids"
  Gain2/1 -> Bus Creator/8  "iqs"
  Hall sensor/1(Hall) -> Demux3/1
  PS-Simulink Converter1/1 -> Phase2neutral/1(vLL)
  Gain6/1 -> Bus Creator/6  "ics"
  Gain5/1 -> Bus Creator/4  "ibs"
  Gain4/1 -> Bus Creator/2  "ias"
  PS-Simulink Converter/1 -> Demux2/1, Park Transform/1
  Te/1 -> Bus Creator/25, Gain12/1  "Electromagnetic torque Te (N*m)"
  Gain12/1 -> Bus Creator/26  "Te"
  Demux3/3 -> Bus Creator/19, Gain11/1  "Hall effect signal h_c"
  Demux3/2 -> Gain10/1, Bus Creator/17  "Hall effect signal h_b"
  Demux3/1 -> Gain9/1, Bus Creator/15  "Hall effect signal h_a"
  thetam/1 -> nPolePairs/1, Gain8/1, Bus Creator/23  "Rotor angle thetam (rad)"
  Bus Creator/1 -> m/1
  Demux2/3 -> Bus Creator/5, Gain6/1  "Stator current is_c (A)"
  Demux2/2 -> Gain5/1, Bus Creator/3  "Stator current is_b (A)"
  Demux2/1 -> Gain4/1, Bus Creator/1  "Stator current is_a (A)"
  Demux1/2 -> Gain3/1, Bus Creator/9  "Stator current is_d (A)"
  Park Transform/1 -> Selector/1
  Demux1/1 -> Gain2/1, Bus Creator/7  "Stator current is_q (A)"
  Demux4/2 -> Gain1/1, Bus Creator/13  "Stator voltage Vs_d (V)"
  Demux4/1 -> Gain/1, Bus Creator/11  "Stator voltage Vs_q (V)"
  Park Transform1/1 -> Selector1/1
  nPolePairs/1 -> Hall sensor/1(thetae), Park Transform1/2, Park Transform/2
  wm/1 -> Bus Creator/21, Gain7/1  "Rotor speed wm (rad/s)"
  connections:
  PS-Simulink Converter1/LConn1 -- Line Voltage Sensor (Three-Phase)/RConn1
  PS-Simulink Converter/LConn1 -- Current Sensor/RConn1
  ~2/RConn1 -- Line Voltage Sensor (Three-Phase)/LConn1 -- Current Sensor/RConn2
  Current Sensor/LConn1 -- ~1/RConn1

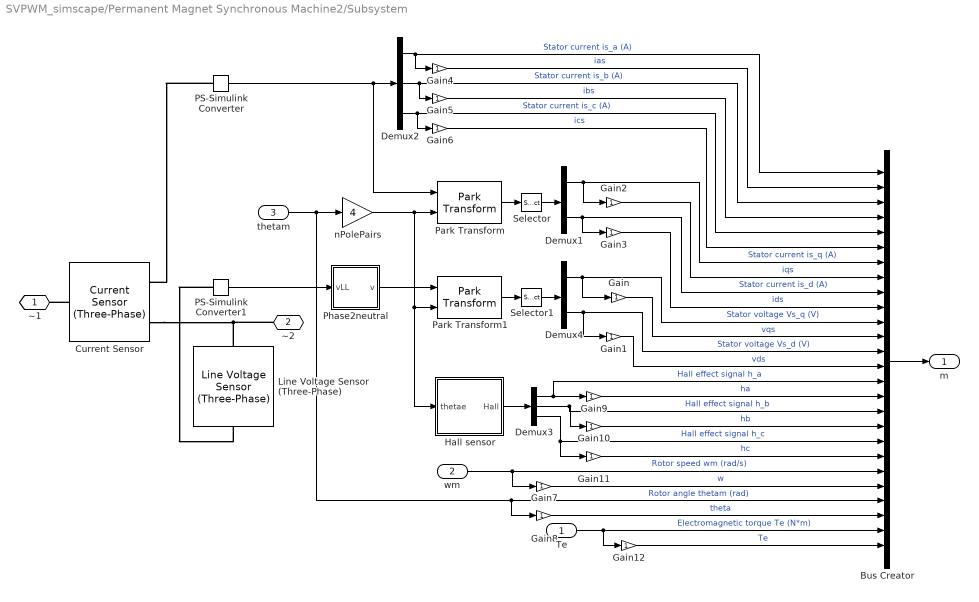
== system SVPWM_simscape/Permanent Magnet Synchronous Machine2/Subsystem ==
  Te : Inport
  wm : Inport  Port=2
  thetam : Inport  Port=3
  Bus Creator : BusCreator  Inputs=26
  Current Sensor : ee_lib/Sensors & Transducers/Current Sensor (Three-Phase)  port_option=ee.enum.threePhasePort.composite
  Demux1 : Demux  Outputs=2
  Demux2 : Demux  Outputs=3
  Demux3 : Demux  Outputs=3
  Demux4 : Demux  Outputs=2
  Gain{,1..12} (13 alike) : Gain
  Hall sensor : Subsystem
  Line Voltage Sensor (Three-Phase) : ee_lib/Sensors & Transducers/Line Voltage Sensor (Three-Phase)  port_option=ee.enum.threePhasePort.composite
  PS-Simulink Converter : nesl_utility/PS-Simulink Converter  PhysicalDomain=network_engine_domain  SubClassName=ps_output  LeftPortType=input  RightPortType=output  PseudoPeriodic=off  Frequencies=[]  VectorFormat=1-D array  Unit=1  AffineConversion=off
  PS-Simulink Converter1 : nesl_utility/PS-Simulink Converter  PhysicalDomain=network_engine_domain  SubClassName=ps_output  LeftPortType=input  RightPortType=output  PseudoPeriodic=off  Frequencies=[]  VectorFormat=1-D array  Unit=1  AffineConversion=off
  Park Transform : eeTransforms/Park Transform  AxisAlignment=D-axis  PowerInvariant=off
  Park Transform1 : eeTransforms/Park Transform  AxisAlignment=D-axis  PowerInvariant=off
  Phase2neutral : Subsystem
  Selector : Selector  InputPortWidth=3  IndexOptions=Index vector (dialog)  Indices=[2 1]  OutputSizes=1
  Selector1 : Selector  InputPortWidth=3  IndexOptions=Index vector (dialog)  Indices=[2 1]  OutputSizes=1
  nPolePairs : Gain  Gain=4
  ~1 : PMIOPort  Side=Left
  ~2 : PMIOPort  Port=2  Side=Right
  m : Outport  VectorParamsAs1DForOutWhenUnconnected=off
  wires:
  Phase2neutral/1(v) -> Park Transform1/1
  Gain8/1 -> Bus Creator/24  "theta"
  Gain7/1 -> Bus Creator/22  "w"
  Selector1/1 -> Demux4/1
  Selector/1 -> Demux1/1
  Gain11/1 -> Bus Creator/20  "hc"
  Gain10/1 -> Bus Creator/18  "hb"
  Gain9/1 -> Bus Creator/16  "ha"
  Gain1/1 -> Bus Creator/14  "vds"
  Gain/1 -> Bus Creator/12  "vqs"
  Gain3/1 -> Bus Creator/10  "ids"
  Gain2/1 -> Bus Creator/8  "iqs"
  Hall sensor/1(Hall) -> Demux3/1
  PS-Simulink Converter1/1 -> Phase2neutral/1(vLL)
  Gain6/1 -> Bus Creator/6  "ics"
  Gain5/1 -> Bus Creator/4  "ibs"
  Gain4/1 -> Bus Creator/2  "ias"
  PS-Simulink Converter/1 -> Demux2/1, Park Transform/1
  Te/1 -> Bus Creator/25, Gain12/1  "Electromagnetic torque Te (N*m)"
  Gain12/1 -> Bus Creator/26  "Te"
  Demux3/3 -> Bus Creator/19, Gain11/1  "Hall effect signal h_c"
  Demux3/2 -> Gain10/1, Bus Creator/17  "Hall effect signal h_b"
  Demux3/1 -> Gain9/1, Bus Creator/15  "Hall effect signal h_a"
  thetam/1 -> nPolePairs/1, Gain8/1, Bus Creator/23  "Rotor angle thetam (rad)"
  Bus Creator/1 -> m/1
  Demux2/3 -> Bus Creator/5, Gain6/1  "Stator current is_c (A)"
  Demux2/2 -> Gain5/1, Bus Creator/3  "Stator current is_b (A)"
  Demux2/1 -> Gain4/1, Bus Creator/1  "Stator current is_a (A)"
  Demux1/2 -> Gain3/1, Bus Creator/9  "Stator current is_d (A)"
  Park Transform/1 -> Selector/1
  Demux1/1 -> Gain2/1, Bus Creator/7  "Stator current is_q (A)"
  Demux4/2 -> Gain1/1, Bus Creator/13  "Stator voltage Vs_d (V)"
  Demux4/1 -> Gain/1, Bus Creator/11  "Stator voltage Vs_q (V)"
  Park Transform1/1 -> Selector1/1
  nPolePairs/1 -> Hall sensor/1(thetae), Park Transform1/2, Park Transform/2
  wm/1 -> Bus Creator/21, Gain7/1  "Rotor speed wm (rad/s)"
  connections:
  PS-Simulink Converter1/LConn1 -- Line Voltage Sensor (Three-Phase)/RConn1
  PS-Simulink Converter/LConn1 -- Current Sensor/RConn1
  ~2/RConn1 -- Line Voltage Sensor (Three-Phase)/LConn1 -- Current Sensor/RConn2
  Current Sensor/LConn1 -- ~1/RConn1

== system SVPWM_simscape/SVPWM计算法/反DQZ变换 ==
  In1 : Inport
  In2 : Inport  Port=2
  In3 : Inport  Port=3
  Bus Creator : BusCreator  Inputs=3
  Fcn : Fcn  Expr=cos(u(3))*u(1)-sin(u(3))*u(2)
  Fcn1 : Fcn  Expr=cos(u(3)-(2*pi/3))*u(1)-sin(u(3)-(2*pi/3))*u(2)
  Fcn2 : Fcn  Expr=cos(u(3)+(2*pi/3))*u(1)-sin(u(3)+(2*pi/3))*u(2)
  A : Outport
  B : Outport  Port=2
  C : Outport  Port=3
  wires:
  In3/1 -> Bus Creator/3  "θe"
  In2/1 -> Bus Creator/2  "Q"
  In1/1 -> Bus Creator/1  "D"
  Bus Creator/1 -> Fcn/1, Fcn1/1, Fcn2/1
  Fcn/1 -> A/1
  Fcn1/1 -> B/1
  Fcn2/1 -> C/1

== system SVPWM_simscape/SVPWM计算法/零序分量计算 ==
  A : Inport
  B : Inport  Port=2
  C : Inport  Port=3
  Gain : Gain  Gain=-0.5
  MinMax : MinMax  Inputs=3
  MinMax1 : MinMax  Function=max  Inputs=3
  Scope : Scope  NumInputPorts=2
      settings: ActiveDisplayYMinimum=-3.75  ActiveDisplayYMaximum=3.75  DataLoggingVariableName=ScopeData3
  Sum : Sum
  Out1 : Outport
  wires:
  A/1 -> MinMax/1, MinMax1/1  "A"
  B/1 -> MinMax1/2, MinMax/2  "B"
  C/1 -> MinMax/3, MinMax1/3  "C"
  MinMax/1 -> Sum/1, Scope/1
  MinMax1/1 -> Scope/2, Sum/2
  Sum/1 -> Gain/1
  Gain/1 -> Out1/1  "V0"

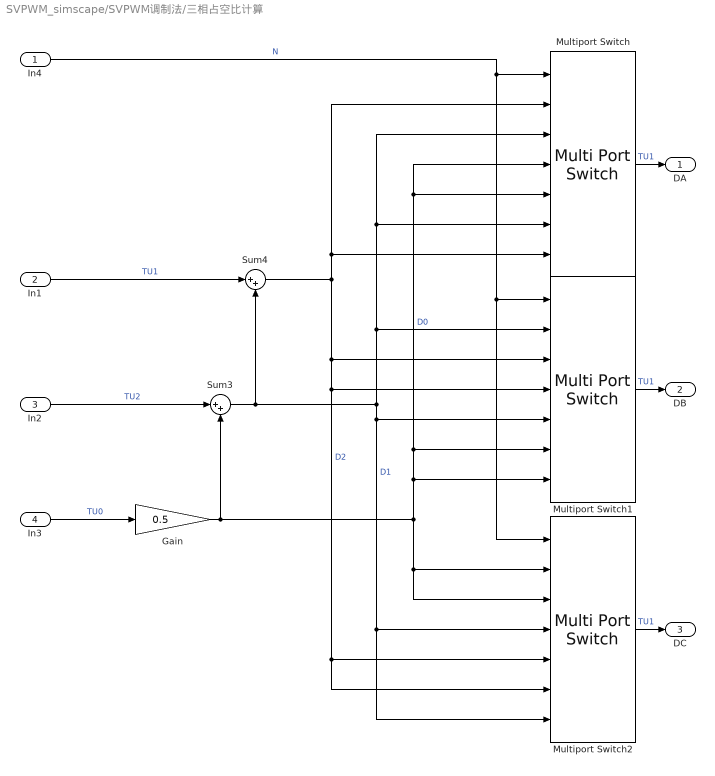
== system SVPWM_simscape/SVPWM调制法/三相占空比计算 ==
  In4 : Inport
  In1 : Inport  Port=2
  In2 : Inport  Port=3
  In3 : Inport  Port=4
  Gain : Gain  Gain=0.5
  Multiport Switch : MultiPortSwitch  Inputs=6  SaturateOnIntegerOverflow=off  InputSameDT=off
  Multiport Switch1 : MultiPortSwitch  Inputs=6  SaturateOnIntegerOverflow=off  InputSameDT=off
  Multiport Switch2 : MultiPortSwitch  Inputs=6  SaturateOnIntegerOverflow=off  InputSameDT=off
  Sum3 : Sum  Inputs=|++
  Sum4 : Sum  Inputs=|++
  DA : Outport
  DB : Outport  Port=2
  DC : Outport  Port=3
  wires:
  Multiport Switch/1 -> DA/1  "TU1"
  Multiport Switch1/1 -> DB/1  "TU1"
  Multiport Switch2/1 -> DC/1  "TU1"
  In3/1 -> Gain/1  "TU0"
  In2/1 -> Sum3/1  "TU2"
  Sum3/1 -> Multiport Switch2/7, Multiport Switch2/4, Multiport Switch1/5, Multiport Switch1/2, Multiport Switch/3, Multiport Switch/6, Sum4/2  "D1"
  In1/1 -> Sum4/1  "TU1"
  In4/1 -> Multiport Switch/1, Multiport Switch1/1, Multiport Switch2/1  "N"
  Sum4/1 -> Multiport Switch2/6, Multiport Switch2/5, Multiport Switch1/4, Multiport Switch1/3, Multiport Switch/7, Multiport Switch/2  "D2"
  Gain/1 -> Multiport Switch1/7, Multiport Switch/5, Multiport Switch/4, Multiport Switch1/6, Multiport Switch2/2, Multiport Switch2/3, Sum3/2  "D0"

== system SVPWM_simscape/SVPWM调制法/反帕克变换 ==
  In1 : Inport
  In2 : Inport  Port=2
  In3 : Inport  Port=3
  Bus Creator : BusCreator  Inputs=3
  Fcn2 : Fcn  Expr=u(1)*cos(u(3))- u(2)*sin(u(3))
  Fcn3 : Fcn  Expr=u(1)*sin(u(3)) + u(2)*cos(u(3))
  A : Outport
  beta : Outport  Port=2
  wires:
  In3/1 -> Bus Creator/3  "θe"
  In2/1 -> Bus Creator/2  "Q"
  In1/1 -> Bus Creator/1  "D"
  Bus Creator/1 -> Fcn2/1, Fcn3/1
  Fcn3/1 -> beta/1  "β"
  Fcn2/1 -> A/1  "α"

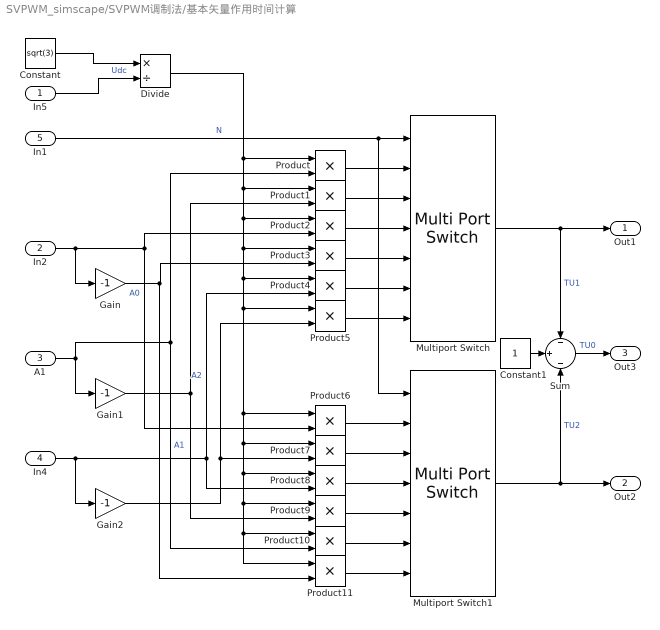
== system SVPWM_simscape/SVPWM调制法/基本矢量作用时间计算 ==
  In5 : Inport
  In2 : Inport  Port=2
  A1 : Inport  Port=3
  In4 : Inport  Port=4
  In1 : Inport  Port=5
  Constant : Constant  Value=sqrt(3)
  Constant1 : Constant
  Divide : Product  Inputs=*/
  Gain : Gain  Gain=-1
  Gain1 : Gain  Gain=-1
  Gain2 : Gain  Gain=-1
  Multiport Switch : MultiPortSwitch  Inputs=6  SaturateOnIntegerOverflow=off  InputSameDT=off
  Multiport Switch1 : MultiPortSwitch  Inputs=6  SaturateOnIntegerOverflow=off  InputSameDT=off
  Product{,1..11} (12 alike) : Product
  Sum : Sum  Inputs=-|+|-
  Out1 : Outport
  Out2 : Outport  Port=2
  Out3 : Outport  Port=3
  wires:
  In1/1 -> Multiport Switch1/1, Multiport Switch/1  "N"
  Multiport Switch1/1 -> Sum/3, Out2/1  "TU2"
  Multiport Switch/1 -> Sum/1, Out1/1  "TU1"
  In5/1 -> Divide/2  "Udc"
  Constant/1 -> Divide/1
  Product/1 -> Multiport Switch/2
  Product5/1 -> Multiport Switch/7
  Product4/1 -> Multiport Switch/6
  Product3/1 -> Multiport Switch/5
  Product2/1 -> Multiport Switch/4
  Product1/1 -> Multiport Switch/3
  Divide/1 -> Product/1, Product6/1, Product11/1, Product10/1, Product9/1, Product8/1, Product7/1, Product5/1, Product4/1, Product3/1, Product2/1, Product1/1
  Product6/1 -> Multiport Switch1/2
  Product7/1 -> Multiport Switch1/3
  Product8/1 -> Multiport Switch1/4
  Product9/1 -> Multiport Switch1/5
  Product10/1 -> Multiport Switch1/6
  Product11/1 -> Multiport Switch1/7
  In2/1 -> Gain/1, Product6/2, Product2/2  "A0"
  A1/1 -> Product10/2, Product/2, Gain1/1  "A1"
  In4/1 -> Product4/2, Product8/2, Gain2/1  "A2"
  Gain1/1 -> Product9/2, Product1/2
  Gain/1 -> Product11/2, Product3/2
  Gain2/1 -> Product7/2, Product5/2
  Sum/1 -> Out3/1  "TU0"
  Constant1/1 -> Sum/2

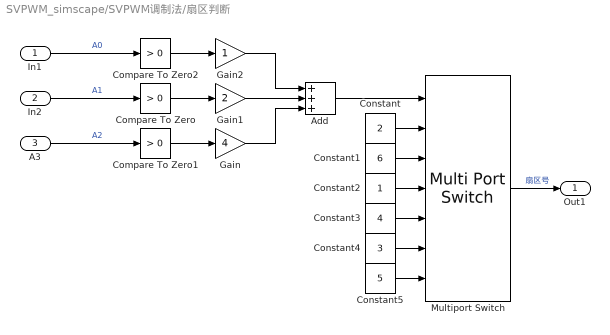
== system SVPWM_simscape/SVPWM调制法/扇区判断 ==
  In1 : Inport
  In2 : Inport  Port=2
  A3 : Inport  Port=3
  Add : Sum  Inputs=+++
  Compare To Zero : simulink/Logic and Bit Operations/Compare To Zero  relop=>  OutDataTypeStr=boolean
  Compare To Zero1 : simulink/Logic and Bit Operations/Compare To Zero  relop=>  OutDataTypeStr=boolean
  Compare To Zero2 : simulink/Logic and Bit Operations/Compare To Zero  relop=>  OutDataTypeStr=boolean
  Constant : Constant  Value=2
  Constant1 : Constant  Value=6
  Constant2 : Constant
  Constant3 : Constant  Value=4
  Constant4 : Constant  Value=3
  Constant5 : Constant  Value=5
  Gain : Gain  Gain=4
  Gain1 : Gain  Gain=2
  Gain2 : Gain
  Multiport Switch : MultiPortSwitch  Inputs=6  SaturateOnIntegerOverflow=off  InputSameDT=off
  Out1 : Outport
  wires:
  In1/1 -> Compare To Zero2/1  "A0"
  In2/1 -> Compare To Zero/1  "A1"
  A3/1 -> Compare To Zero1/1  "A2"
  Compare To Zero2/1 -> Gain2/1
  Compare To Zero/1 -> Gain1/1
  Compare To Zero1/1 -> Gain/1
  Gain2/1 -> Add/1
  Gain1/1 -> Add/2
  Gain/1 -> Add/3
  Add/1 -> Multiport Switch/1
  Constant/1 -> Multiport Switch/2
  Constant1/1 -> Multiport Switch/3
  Constant2/1 -> Multiport Switch/4
  Constant3/1 -> Multiport Switch/5
  Constant4/1 -> Multiport Switch/6
  Constant5/1 -> Multiport Switch/7
  Multiport Switch/1 -> Out1/1  "扇区号"

== system SVPWM_simscape/SVPWM调制法/逻辑向量计算 ==
  A : Inport
  beta : Inport  Port=2
  Bus Creator : BusCreator  Inputs=3
  Fcn : Fcn  Expr=u(3)
  Fcn1 : Fcn  Expr=sqrt(3)/2*u(2)-0.5*u(3)
  Fcn2 : Fcn  Expr=-sqrt(3)/2*u(2)-0.5*u(3)
  Out1 : Outport
  Out2 : Outport  Port=2
  Out3 : Outport  Port=3
  wires:
  A/1 -> Bus Creator/2  "α"
  beta/1 -> Bus Creator/3  "β"
  ? -> Bus Creator/1  "U_dc"
  Bus Creator/1 -> Fcn2/1, Fcn1/1, Fcn/1
  Fcn/1 -> Out1/1  "A0"
  Fcn1/1 -> Out2/1  "A1"
  Fcn2/1 -> Out3/1  "A2"
